simulink model "three_time_scale"  (R2015b)
settings: Solver=ode45  StartTime=0.0  StopTime=50000.0  RelTol=1e-3
values from neighbouring files (symbols this model uses):
  alpha = a(i)    [AsymOscillPeriods.m]    (also in averagedRelayOutput.m = alphaArray(i); bursting_linearised.m = 0.5; compareApproximations.m = 0.5; evaluateDerivatives.m = variables(3))
  beta = 0.37    [averagedRelayOutput.m]    (also in bursting_linearised.m = 0.27; compareApproximations.m = 1.5; fastSlow.m; fast_nullcline_winged_cusp.m = 0.5)
  delta = 0.5    [averagedRelayOutput.m]    (also in bursting_linearised.m; compareApproximations.m; fastSlow.m; fast_nullcline_winged_cusp.m)
  fast_plant_X0 = -1.0    (= -1)    [averagedRelayOutput.m]    (also in bursting_linearised.m = -1.05; fastSlow.m; fast_nullcline_winged_cusp.m; hRose.m = 0)
  gamma = 0    [averagedRelayOutput.m]    (also in bursting_linearised.m = 1; compareApproximations.m = 1; fastSlow.m; fast_nullcline_winged_cusp.m = 1)
  slow_plant_X0 = -1.0    (= -1)    [averagedRelayOutput.m]    (also in bursting_linearised.m = -1.05; fastSlow.m; fast_nullcline_winged_cusp.m = -2; hRose.m = -10)
  ts = 1    [averagedRelayOutput.m]    (also in bursting_linearised.m; compareApproximations.m; fastSlow.m; fast_nullcline_winged_cusp.m)
libraries: simulink x1
settings Model: Creator=rajiv  LastModifiedBy=rajiv
settings HardwareCC: ProdWordSize=32  ProdHWDeviceType=Specified

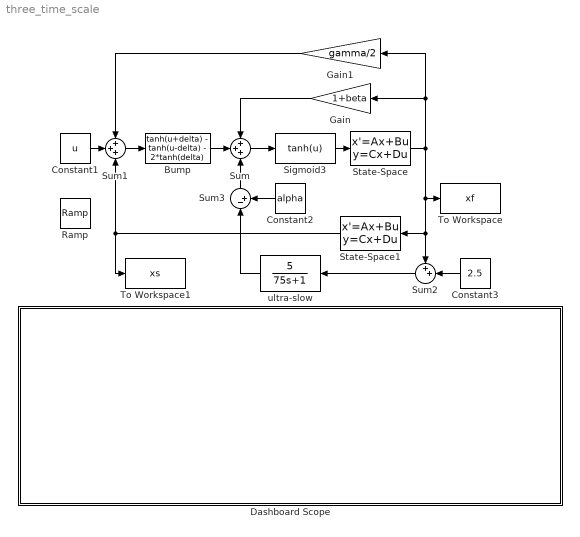
== system three_time_scale ==
  Bump : Fcn  Expr="tanh(u+delta) -  tanh(u-delta) - 2*tanh(delta)"
  Constant1 : Constant  Value=u
  Constant2 : Constant  Value=alpha
  Constant3 : Constant  Value=2.5
  Dashboard Scope : Subsystem  DialogController=hmiCreateDDGDialog  IsWebBlock=on  mask(MWDashboardBlock){webBlockId=8879f959-95f0-45f4-b2bb-9dff7a2f39be, webBlockType=sdiscope, ShowInitialText=on, HMISrcModelName=three_time_scale}
      mask prompts: webBlockId "WebBlock Id"; webBlockType "WebBlock Type"; HMISrcModelName "Source Model"
      mask Help: helpview([docroot '/mapfiles/simulink.map'], 'hmi_scope')
      mask Display:
      | if strcmp(get_param(bdroot(gcb),'BlockDiagramType'), 'library')
      |     image([(matlabroot) '/toolbox/simulink/hmi/icons/DashboardScope.png']);
      | end
  Gain : Gain  Gain=1+beta
  Gain1 : Gain  Gain=gamma/2
  Ramp : simulink/Sources/Ramp  slope=6e-5  start=0  X0=0
  Sigmoid3 : Fcn  Expr=tanh(u)
  State-Space : StateSpace  A=-1/tf  B=1/tf  D=0  X0=fast_plant_X0
  State-Space1 : StateSpace  A=-1/ts  B=1/ts  D=0  X0=slow_plant_X0
  Sum : Sum  Inputs=+++
  Sum1 : Sum  Inputs=+++
  Sum2 : Sum  Inputs=++|
  Sum3 : Sum  Inputs=|-+
  To Workspace : ToWorkspace  VariableName=xf  SaveFormat=Timeseries  SampleTime=-1
  To Workspace1 : ToWorkspace  VariableName=xs  SaveFormat=Timeseries  SampleTime=-1
  ultra-slow : TransferFcn  Numerator=[5]  Denominator=[75 1]
  wires:
  Sum/1 -> Sigmoid3/1
  Gain/1 -> Sum/1
  State-Space1/1 -> Sum1/3, To Workspace1/1
  Gain1/1 -> Sum1/1
  Sigmoid3/1 -> State-Space/1
  State-Space/1 -> Gain/1, Gain1/1, To Workspace/1, Sum2/1, State-Space1/1
  Sum3/1 -> Sum/3
  Constant2/1 -> Sum3/2
  ultra-slow/1 -> Sum3/1
  Sum2/1 -> ultra-slow/1
  Constant3/1 -> Sum2/2
  Constant1/1 -> Sum1/2
  Sum1/1 -> Bump/1
  Bump/1 -> Sum/2

== system three_time_scale/Dashboard Scope ==
